simulink model "DC_Motor_controller"  (Simulink 7.5)
settings: Solver=ode45  StartTime=0.0  StopTime=10  RelTol=1e-3
values from neighbouring files (symbols this model uses):
  J = 52E-7    (= 5.2e-06)    [DesignDCMotorUsingPIDrlocusBode.m]    (also in DiscreteDesignandEquivalent.m; bode_mcode.m; il_zom_hae_byungsina.m; rlocus_mcode.m)
  Ra = zeros(1,180)    [AccelandBrake1.m]
undefined symbols (not defined in the file or in its folder): B, Ke, Kt, La
settings Model: Creator=page365  LastModifiedBy=page365

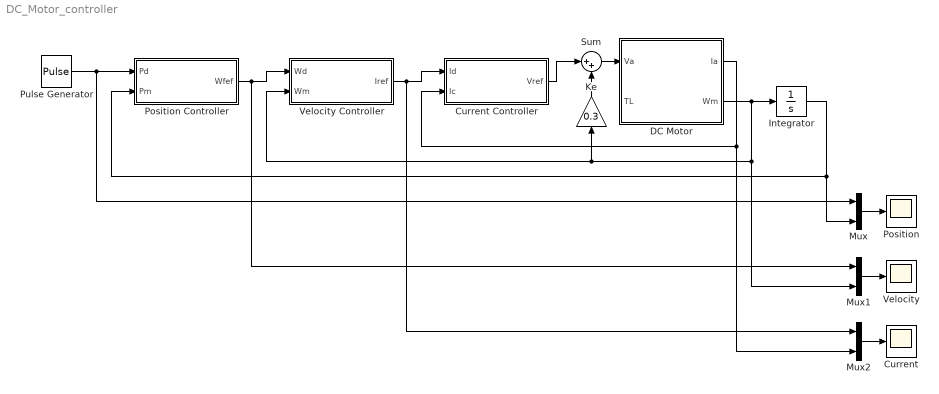
== system DC_Motor_controller ==
  Current : Scope
      settings: TimeRange=10  YMin=-20  YMax=20  SaveName=ScopeData2
  Current Controller : Subsystem
  DC Motor : Subsystem
  Integrator : Integrator
  Ke : Gain  Gain=0.3  ParameterDataType=fixdt(1, 16)  ParameterScaling=2^0  OutDataType=fixdt(1, 16)  OutScaling=2^0
  Mux : Mux  Inputs=2
  Mux1 : Mux  Inputs=2
  Mux2 : Mux  Inputs=2
  Position : Scope
      settings: TimeRange=10  YMin=0  YMax=150
  Position Controller : Subsystem
  Pulse Generator : DiscretePulseGenerator  PulseType=Time based  Amplitude=100  Period=10  PulseWidth=50  PhaseDelay=1  SampleTime=1
  Sum : Sum  Inputs=|++  OutDataType=fixdt(1, 16)  OutScaling=2^0
  Velocity : Scope
      settings: TimeRange=10  YMin=-100  YMax=100
  Velocity Controller : Subsystem
  wires:
  Mux/1 -> Position/1
  DC Motor/1(Ia) -> Current Controller/2(Ic), Mux2/2
  Velocity Controller/1(Iref) -> Current Controller/1(Id), Mux2/1
  DC Motor/2(Wm) -> Integrator/1, Mux1/2, Velocity Controller/2(Wm), Ke/1
  Integrator/1 -> Position Controller/2(Pm), Mux/2
  Position Controller/1(Wfef) -> Velocity Controller/1(Wd), Mux1/1
  Pulse Generator/1 -> Position Controller/1(Pd), Mux/1
  Mux1/1 -> Velocity/1
  Mux2/1 -> Current/1
  Current Controller/1(Vref) -> Sum/1
  Sum/1 -> DC Motor/1(Va)
  Ke/1 -> Sum/2

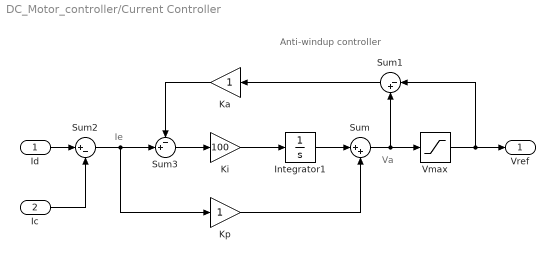
== system DC_Motor_controller/Current Controller ==
  note: Anti-windup controller
  note: Ie
  note: Va
  Id : Inport  OutDataType=fixdt(1, 16)  OutScaling=2^0
  Ic : Inport  Port=2  OutDataType=fixdt(1, 16)  OutScaling=2^0
  Integrator1 : Integrator
  Ka : Gain  ParameterDataType=fixdt(1, 16)  ParameterScaling=2^0  OutDataType=fixdt(1, 16)  OutScaling=2^0
  Ki : Gain  Gain=100  ParameterDataType=fixdt(1, 16)  ParameterScaling=2^0  OutDataType=fixdt(1, 16)  OutScaling=2^0
  Kp : Gain  ParameterDataType=fixdt(1, 16)  ParameterScaling=2^0  OutDataType=fixdt(1, 16)  OutScaling=2^0
  Sum : Sum  Inputs=|++  OutDataType=fixdt(1, 16)  OutScaling=2^0
  Sum1 : Sum  Inputs=|-+  OutDataType=fixdt(1, 16)  OutScaling=2^0
  Sum2 : Sum  Inputs=|+-  OutDataType=fixdt(1, 16)  OutScaling=2^0
  Sum3 : Sum  Inputs=-+|  OutDataType=fixdt(1, 16)  OutScaling=2^0
  Vmax : Saturate  UpperLimit=20  LowerLimit=-20  OutDataType=fixdt(1, 16)  OutScaling=2^0
  Vref : Outport  OutDataType=fixdt(1, 16)  OutScaling=2^0
  wires:
  Vmax/1 -> Sum1/1, Vref/1
  Kp/1 -> Sum/2
  Integrator1/1 -> Sum/1
  Ki/1 -> Integrator1/1
  Sum/1 -> Vmax/1, Sum1/2
  Sum1/1 -> Ka/1
  Ka/1 -> Sum3/1
  Sum3/1 -> Ki/1
  Sum2/1 -> Sum3/2, Kp/1
  Id/1 -> Sum2/1
  Ic/1 -> Sum2/2

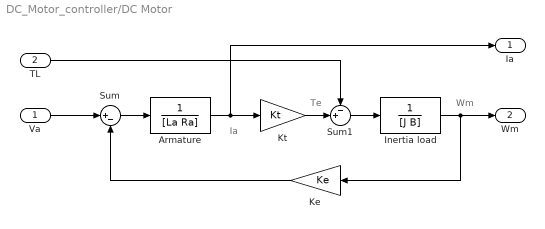
== system DC_Motor_controller/DC Motor ==
  note: Ia
  note: Te
  note: Wm
  Va : Inport  OutDataType=fixdt(1, 16)  OutScaling=2^0
  TL : Inport  Port=2  OutDataType=fixdt(1, 16)  OutScaling=2^0
  Armature : TransferFcn  Denominator=[La Ra]
  Inertia load : TransferFcn  Denominator=[J B]
  Ke : Gain  Gain=Ke  ParameterDataType=fixdt(1, 16)  ParameterScaling=2^0  OutDataType=fixdt(1, 16)  OutScaling=2^0
  Kt : Gain  Gain=Kt  ParameterDataType=fixdt(1, 16)  ParameterScaling=2^0  OutDataType=fixdt(1, 16)  OutScaling=2^0
  Sum : Sum  Inputs=|+-  OutDataType=fixdt(1, 16)  OutScaling=2^0
  Sum1 : Sum  Inputs=-+|  OutDataType=fixdt(1, 16)  OutScaling=2^0
  Ia : Outport  OutDataType=fixdt(1, 16)  OutScaling=2^0
  Wm : Outport  Port=2  OutDataType=fixdt(1, 16)  OutScaling=2^0
  wires:
  Inertia load/1 -> Ke/1, Wm/1
  Sum1/1 -> Inertia load/1
  Armature/1 -> Kt/1, Ia/1
  Sum/1 -> Armature/1
  Ke/1 -> Sum/2
  Va/1 -> Sum/1
  TL/1 -> Sum1/1
  Kt/1 -> Sum1/2

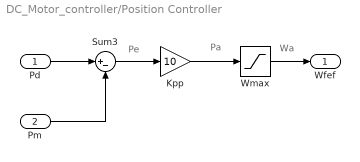
== system DC_Motor_controller/Position Controller ==
  note: Pe
  note: Pa
  note: Wa
  Pd : Inport  OutDataType=fixdt(1, 16)  OutScaling=2^0
  Pm : Inport  Port=2  OutDataType=fixdt(1, 16)  OutScaling=2^0
  Kpp : Gain  Gain=10  ParameterDataType=fixdt(1, 16)  ParameterScaling=2^0  OutDataType=fixdt(1, 16)  OutScaling=2^0
  Sum3 : Sum  Inputs=|+-  OutDataType=fixdt(1, 16)  OutScaling=2^0
  Wmax : Saturate  UpperLimit=100  LowerLimit=-100  OutDataType=fixdt(1, 16)  OutScaling=2^0
  Wfef : Outport  OutDataType=fixdt(1, 16)  OutScaling=2^0
  wires:
  Kpp/1 -> Wmax/1
  Pd/1 -> Sum3/1
  Sum3/1 -> Kpp/1
  Pm/1 -> Sum3/2
  Wmax/1 -> Wfef/1

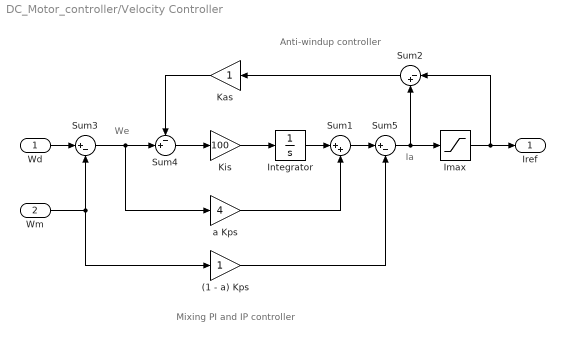
== system DC_Motor_controller/Velocity Controller ==
  note: Mixing PI and IP controller
  note: Anti-windup controller
  note: Ia
  note: We
  Wd : Inport  OutDataType=fixdt(1, 16)  OutScaling=2^0
  Wm : Inport  Port=2  OutDataType=fixdt(1, 16)  OutScaling=2^0
  (1 - a) Kps : Gain  ParameterDataType=fixdt(1, 16)  ParameterScaling=2^0  OutDataType=fixdt(1, 16)  OutScaling=2^0
  Imax : Saturate  UpperLimit=20  LowerLimit=-20  OutDataType=fixdt(1, 16)  OutScaling=2^0
  Integrator : Integrator
  Kas : Gain  ParameterDataType=fixdt(1, 16)  ParameterScaling=2^0  OutDataType=fixdt(1, 16)  OutScaling=2^0
  Kis : Gain  Gain=100  ParameterDataType=fixdt(1, 16)  ParameterScaling=2^0  OutDataType=fixdt(1, 16)  OutScaling=2^0
  Sum1 : Sum  Inputs=|++  OutDataType=fixdt(1, 16)  OutScaling=2^0
  Sum2 : Sum  Inputs=|-+  OutDataType=fixdt(1, 16)  OutScaling=2^0
  Sum3 : Sum  Inputs=|+-  OutDataType=fixdt(1, 16)  OutScaling=2^0
  Sum4 : Sum  Inputs=-+|  OutDataType=fixdt(1, 16)  OutScaling=2^0
  Sum5 : Sum  Inputs=|+-  OutDataType=fixdt(1, 16)  OutScaling=2^0
  a Kps : Gain  Gain=4  ParameterDataType=fixdt(1, 16)  ParameterScaling=2^0  OutDataType=fixdt(1, 16)  OutScaling=2^0
  Iref : Outport  OutDataType=fixdt(1, 16)  OutScaling=2^0
  wires:
  Kis/1 -> Integrator/1
  Sum3/1 -> a Kps/1, Sum4/2
  Wd/1 -> Sum3/1
  Wm/1 -> Sum3/2, (1 - a) Kps/1
  Sum5/1 -> Imax/1, Sum2/2
  Imax/1 -> Iref/1, Sum2/1
  Sum2/1 -> Kas/1
  Kas/1 -> Sum4/1
  Sum4/1 -> Kis/1
  Sum1/1 -> Sum5/1
  Integrator/1 -> Sum1/1
  a Kps/1 -> Sum1/2
  (1 - a) Kps/1 -> Sum5/2
